simulink library "windFrameToTangentialPlaneKinVel_ul"  (R2018b)
settings: Solver=VariableStepAuto  StartTime=0.0  StopTime=10.0  RelTol=1e-3
values from neighbouring files (symbols this model uses):
  V = [-sin(phi1).*cos(lambda1), -sin(lambda1) ... (first row only)    [plotFigure8.m]
libraries: dspinverses x1
settings Model: Creator=James Reed  LastModifiedBy=James Reed

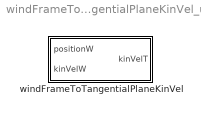
== system windFrameToTangentialPlaneKinVel_ul ==
  windFrameToTangentialPlaneKinVel : Subsystem

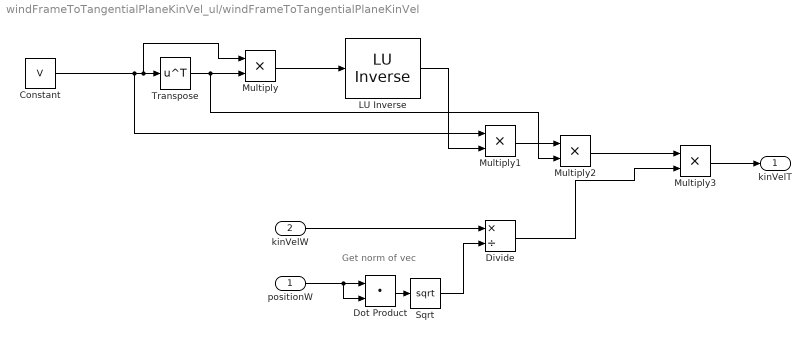
== system windFrameToTangentialPlaneKinVel_ul/windFrameToTangentialPlaneKinVel ==
  note: Get norm of vec
  positionW : Inport
  kinVelW : Inport  Port=2
  " LU Inverse" : dspinverses/ LU Inverse
      settings: SourceProductName=DSP System Toolbox
  Constant : Constant  Value=V
  Divide : Product  Inputs=*/
  Dot Product : DotProduct  InputSameDT=on  OutDataTypeStr=Inherit: Inherit via internal rule
  Multiply{,1..3} (4 alike) : Product
  Sqrt : Sqrt  SaturateOnIntegerOverflow=on
  Transpose : Math  Operator=transpose  SaturateOnIntegerOverflow=on
  kinVelT : Outport
  wires:
  Transpose/1 -> Multiply2/2, Multiply/2
  Multiply2/1 -> Multiply3/1
  " LU Inverse"/1 -> Multiply1/2
  positionW/1 -> Dot Product/2, Dot Product/1
  Multiply/1 -> " LU Inverse"/1
  Multiply1/1 -> Multiply2/1
  Multiply3/1 -> kinVelT/1
  Divide/1 -> Multiply3/2
  kinVelW/1 -> Divide/1
  Sqrt/1 -> Divide/2
  Constant/1 -> Multiply1/1, Multiply/1, Transpose/1
  Dot Product/1 -> Sqrt/1
